simulink model "PMSM_FOC_CascadeControl"  (R2026a)
settings: Solver=ode4  StopTime=simulation_stop_time_s  FixedStep=Ts_current
InitFcn:
  | init_pmsm_foc_cascade
values from neighbouring files (symbols this model uses):
  iq_ref_limit_a = 8.0    (= 8)    [init_pmsm_foc_cascade.m]
  Ki_id = 300.0    (= 300)    [init_pmsm_foc_cascade.m]
  Ki_iq = 300.0    (= 300)    [init_pmsm_foc_cascade.m]
  Ki_speed = 4.0    (= 4)    [init_pmsm_foc_cascade.m]
  Kp_id = 1.5    [init_pmsm_foc_cascade.m]
  Kp_iq = 1.5    [init_pmsm_foc_cascade.m]
  Kp_position = 8.0    (= 8)    [init_pmsm_foc_cascade.m]
  Kp_speed = 0.20    (= 0.2)    [init_pmsm_foc_cascade.m]
  load_torque_nm = 0.0    (= 0)    [init_pmsm_foc_cascade.m]
  pmsm_B_nms = 1.0e-5    (= 1e-05)    [init_pmsm_foc_cascade.m]
  pmsm_flux_wb = 6.0e-3    (= 0.006)    [init_pmsm_foc_cascade.m]
  pmsm_J_kg_m2 = 2.0e-5    (= 2e-05)    [init_pmsm_foc_cascade.m]
  pmsm_Ld_h = 2.0e-4    (= 0.0002)    [init_pmsm_foc_cascade.m]
  pmsm_Lq_h = 2.0e-4    (= 0.0002)    [init_pmsm_foc_cascade.m]
  pmsm_pole_pairs = 7    [init_pmsm_foc_cascade.m]
  pmsm_Rs_ohm = 0.30    (= 0.3)    [init_pmsm_foc_cascade.m]
  position_step_time_s = 0.02    [init_pmsm_foc_cascade.m]
  speed_ref_limit_rad_s = 80.0    (= 80)    [init_pmsm_foc_cascade.m]
  Ts_current = 1.0e-4    (= 0.0001)    [init_pmsm_foc_cascade.m]
  Ts_position = Ts_current    (= 0.0001)    [init_pmsm_foc_cascade.m]
  Ts_speed = Ts_current    (= 0.0001)    [init_pmsm_foc_cascade.m]
  Vdc = 12.0    (= 12)    [init_pmsm_foc_cascade.m]
  voltage_limit_v = Vdc / sqrt(3.0)    [init_pmsm_foc_cascade.m]
libraries: slpidlib x3
settings Model: Creator=tgs27  LastModifiedBy=tgs27

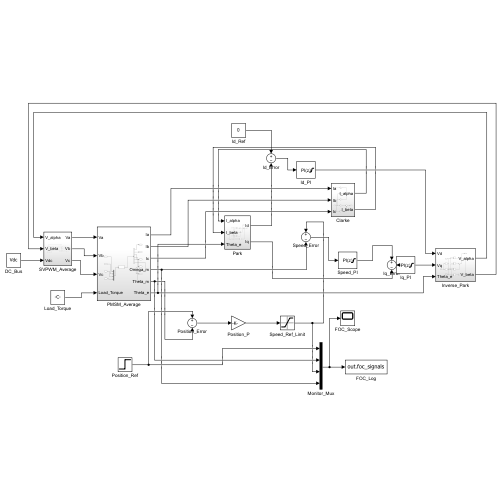
[thumbnail: Simulink's stored preview of the top-level diagram]
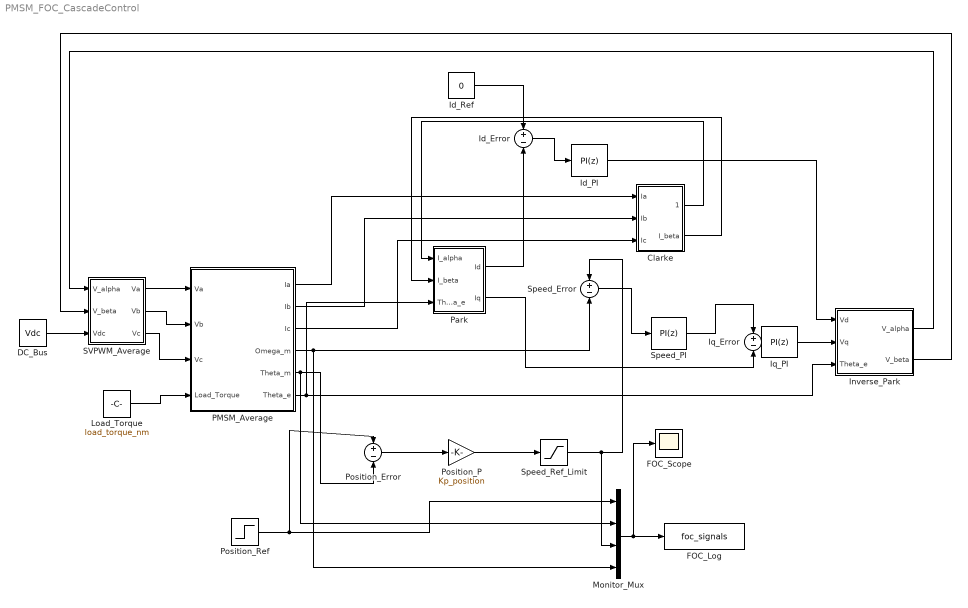
== system PMSM_FOC_CascadeControl ==
  Clarke : Subsystem
  DC_Bus : Constant  Value=Vdc
  FOC_Log : ToWorkspace  VariableName=foc_signals  SaveFormat=Structure With Time
  FOC_Scope : Scope
  Id_Error : Sum  Inputs=+-
  Id_PI : slpidlib/PID Controller  Controller=PI  Form=Parallel  TimeDomain=Discrete-time  UseExternalTs=off  SampleTime=Ts_current  IntegratorMethod=Forward Euler  FilterMethod=Forward Euler  ControllerParametersSource=internal  P=Kp_id  I=Ki_id  UseKiTs=off  D=0  UseExternalDerivativeSource=off  N=100  UseFilter=on  TunerSelectOption=Transfer Function Based (PID Tuner App)  InitialConditionSource=internal  InitialConditionForIntegrator=0  InitialConditionForFilter=0  DifferentiatorICPrevScaledInput=0  ExternalReset=none  TrackingMode=off  Kt=1  LimitOutput=on  SatLimitsSource=internal  UpperSaturationLimit=voltage_limit_v  LowerSaturationLimit=-voltage_limit_v  LinearizeAsGain=on  AntiWindupMode=none  Kb=1  LimitIntegrator=off  UpperIntegratorSaturationLimit=inf  LowerIntegratorSaturationLimit=-inf  POutMin=[]  POutMax=[]  IOutMin=[]  IOutMax=[]  DOutMin=[]  DOutMax=[]  NOutMin=[]  NOutMax=[]  SumOutMin=[]  SumOutMax=[]  SaturationOutMin=[]  SaturationOutMax=[]  PParamMin=[]  PParamMax=[]  IParamMin=[]  IParamMax=[]  DParamMin=[]  DParamMax=[]  NParamMin=[]  NParamMax=[]  KbParamMin=[]  KbParamMax=[]  KtParamMin=[]  KtParamMax=[]  KbOutMin=[]  KbOutMax=[]  KtOutMin=[]  KtOutMax=[]  IntegratorOutMin=[]  IntegratorOutMax=[]  FilterOutMin=[]  FilterOutMax=[]  SumI1OutMin=[]  SumI1OutMax=[]  SumI2OutMin=[]  SumI2OutMax=[]  SumI3OutMin=[]  SumI3OutMax=[]  SumI4OutMin=[]  SumI4OutMax=[]  SumDOutMin=[]  SumDOutMax=[]  DifferentiatorOutMin=[]  DifferentiatorOutMax=[]  FilterDiffOutCoefMin=[]  FilterDiffOutCoefMax=[]  ReciprocalOutMin=[]  ReciprocalOutMax=[]  SumDenOutMin=[]  SumDenOutMax=[]  SumNumOutMin=[]  SumNumOutMax=[]  DivideOutMin=[]  DivideOutMax=[]  UdiffTsProdOutMin=[]  UdiffTsProdOutMax=[]  NTsProdOutMin=[]  NTsProdOutMax=[]  UintegralTsProdOutMin=[]  UintegralTsProdOutMax=[]  UngainTsProdOutMin=[]  UngainTsProdOutMax=[]  ClampingZeroOutDataTypeStr=Inherit: Inherit via back propagation  ClampingZeroOutMin=[]  ClampingZeroOutMax=[]  FilterDenConstantOutDataTypeStr=Inherit: Inherit via back propagation  FilterDenConstantOutMin=[]  FilterDenConstantOutMax=[]  PCopyOutDataTypeStr=Inherit: Inherit via back propagation  PCopyOutMin=[]  PCopyOutMax=[]  NCopyOutDataTypeStr=Inherit: Inherit via back propagation  NCopyOutMin=[]  NCopyOutMax=[]  IntegratorContinuousStateAttributes=''  IntegratorStateMustResolveToSignalObject=off  IntegratorRTWStateStorageClass=Auto  FilterContinuousStateAttributes=''  FilterStateMustResolveToSignalObject=off  FilterRTWStateStorageClass=Auto  ParallelPVariant=InternalParameters  IdealPVariant=Disabled  IVariant=InternalParameters  DVariant=Disabled  IntegratorVariant=Discrete  SatVariant=Enabled  AWVariant=Passthrough  PCopyVariant=Disabled  TRVariant=Disabled  FdbkBlocksVariant=Forward  IdealPFdbkVariant=Disabled  SatFdbkVariant=Disabled  DerivativeFilterVariant=Disabled  NVariant=Disabled  NCopyVariant=Disabled_SignalSpec  FilterICVariant=Disabled  IntegratorICVariant=InternalICs  ExternalResetVariant=Disabled  TRSumVariant=Passthrough  SumFdbkVariant=Disabled  SumVariant=Sum_PI  TsampFilterVariant=InternalTs  TsampNgainVariant=Passthrough  TsampIntegralVariant=Disabled_SignalSpec  ExternalSaturationOutDataTypeStr=Inherit: Same as second input  DerivativeSourceVariant=Disabled  PreIntVariant=InternalPreInt
  Id_Ref : Constant  Value=0
  Inverse_Park : Subsystem
  Iq_Error : Sum  Inputs=+-
  Iq_PI : slpidlib/PID Controller  Controller=PI  Form=Parallel  TimeDomain=Discrete-time  UseExternalTs=off  SampleTime=Ts_current  IntegratorMethod=Forward Euler  FilterMethod=Forward Euler  ControllerParametersSource=internal  P=Kp_iq  I=Ki_iq  UseKiTs=off  D=0  UseExternalDerivativeSource=off  N=100  UseFilter=on  TunerSelectOption=Transfer Function Based (PID Tuner App)  InitialConditionSource=internal  InitialConditionForIntegrator=0  InitialConditionForFilter=0  DifferentiatorICPrevScaledInput=0  ExternalReset=none  TrackingMode=off  Kt=1  LimitOutput=on  SatLimitsSource=internal  UpperSaturationLimit=voltage_limit_v  LowerSaturationLimit=-voltage_limit_v  LinearizeAsGain=on  AntiWindupMode=none  Kb=1  LimitIntegrator=off  UpperIntegratorSaturationLimit=inf  LowerIntegratorSaturationLimit=-inf  POutMin=[]  POutMax=[]  IOutMin=[]  IOutMax=[]  DOutMin=[]  DOutMax=[]  NOutMin=[]  NOutMax=[]  SumOutMin=[]  SumOutMax=[]  SaturationOutMin=[]  SaturationOutMax=[]  PParamMin=[]  PParamMax=[]  IParamMin=[]  IParamMax=[]  DParamMin=[]  DParamMax=[]  NParamMin=[]  NParamMax=[]  KbParamMin=[]  KbParamMax=[]  KtParamMin=[]  KtParamMax=[]  KbOutMin=[]  KbOutMax=[]  KtOutMin=[]  KtOutMax=[]  IntegratorOutMin=[]  IntegratorOutMax=[]  FilterOutMin=[]  FilterOutMax=[]  SumI1OutMin=[]  SumI1OutMax=[]  SumI2OutMin=[]  SumI2OutMax=[]  SumI3OutMin=[]  SumI3OutMax=[]  SumI4OutMin=[]  SumI4OutMax=[]  SumDOutMin=[]  SumDOutMax=[]  DifferentiatorOutMin=[]  DifferentiatorOutMax=[]  FilterDiffOutCoefMin=[]  FilterDiffOutCoefMax=[]  ReciprocalOutMin=[]  ReciprocalOutMax=[]  SumDenOutMin=[]  SumDenOutMax=[]  SumNumOutMin=[]  SumNumOutMax=[]  DivideOutMin=[]  DivideOutMax=[]  UdiffTsProdOutMin=[]  UdiffTsProdOutMax=[]  NTsProdOutMin=[]  NTsProdOutMax=[]  UintegralTsProdOutMin=[]  UintegralTsProdOutMax=[]  UngainTsProdOutMin=[]  UngainTsProdOutMax=[]  ClampingZeroOutDataTypeStr=Inherit: Inherit via back propagation  ClampingZeroOutMin=[]  ClampingZeroOutMax=[]  FilterDenConstantOutDataTypeStr=Inherit: Inherit via back propagation  FilterDenConstantOutMin=[]  FilterDenConstantOutMax=[]  PCopyOutDataTypeStr=Inherit: Inherit via back propagation  PCopyOutMin=[]  PCopyOutMax=[]  NCopyOutDataTypeStr=Inherit: Inherit via back propagation  NCopyOutMin=[]  NCopyOutMax=[]  IntegratorContinuousStateAttributes=''  IntegratorStateMustResolveToSignalObject=off  IntegratorRTWStateStorageClass=Auto  FilterContinuousStateAttributes=''  FilterStateMustResolveToSignalObject=off  FilterRTWStateStorageClass=Auto  ParallelPVariant=InternalParameters  IdealPVariant=Disabled  IVariant=InternalParameters  DVariant=Disabled  IntegratorVariant=Discrete  SatVariant=Enabled  AWVariant=Passthrough  PCopyVariant=Disabled  TRVariant=Disabled  FdbkBlocksVariant=Forward  IdealPFdbkVariant=Disabled  SatFdbkVariant=Disabled  DerivativeFilterVariant=Disabled  NVariant=Disabled  NCopyVariant=Disabled_SignalSpec  FilterICVariant=Disabled  IntegratorICVariant=InternalICs  ExternalResetVariant=Disabled  TRSumVariant=Passthrough  SumFdbkVariant=Disabled  SumVariant=Sum_PI  TsampFilterVariant=InternalTs  TsampNgainVariant=Passthrough  TsampIntegralVariant=Disabled_SignalSpec  ExternalSaturationOutDataTypeStr=Inherit: Same as second input  DerivativeSourceVariant=Disabled  PreIntVariant=InternalPreInt
  Load_Torque : Constant  Value=load_torque_nm
  Monitor_Mux : Mux
  PMSM_Average : Subsystem
  Park : Subsystem
  Position_Error : Sum  Inputs=+-
  Position_P : Gain  Gain=Kp_position
  Position_Ref : Step  Time=position_step_time_s  FinalValue=position_step_rad  SampleTime=Ts_position
  SVPWM_Average : Subsystem
  Speed_Error : Sum  Inputs=+-
  Speed_PI : slpidlib/PID Controller  Controller=PI  Form=Parallel  TimeDomain=Discrete-time  UseExternalTs=off  SampleTime=Ts_speed  IntegratorMethod=Forward Euler  FilterMethod=Forward Euler  ControllerParametersSource=internal  P=Kp_speed  I=Ki_speed  UseKiTs=off  D=0  UseExternalDerivativeSource=off  N=100  UseFilter=on  TunerSelectOption=Transfer Function Based (PID Tuner App)  InitialConditionSource=internal  InitialConditionForIntegrator=0  InitialConditionForFilter=0  DifferentiatorICPrevScaledInput=0  ExternalReset=none  TrackingMode=off  Kt=1  LimitOutput=on  SatLimitsSource=internal  UpperSaturationLimit=iq_ref_limit_a  LowerSaturationLimit=-iq_ref_limit_a  LinearizeAsGain=on  AntiWindupMode=none  Kb=1  LimitIntegrator=off  UpperIntegratorSaturationLimit=inf  LowerIntegratorSaturationLimit=-inf  POutMin=[]  POutMax=[]  IOutMin=[]  IOutMax=[]  DOutMin=[]  DOutMax=[]  NOutMin=[]  NOutMax=[]  SumOutMin=[]  SumOutMax=[]  SaturationOutMin=[]  SaturationOutMax=[]  PParamMin=[]  PParamMax=[]  IParamMin=[]  IParamMax=[]  DParamMin=[]  DParamMax=[]  NParamMin=[]  NParamMax=[]  KbParamMin=[]  KbParamMax=[]  KtParamMin=[]  KtParamMax=[]  KbOutMin=[]  KbOutMax=[]  KtOutMin=[]  KtOutMax=[]  IntegratorOutMin=[]  IntegratorOutMax=[]  FilterOutMin=[]  FilterOutMax=[]  SumI1OutMin=[]  SumI1OutMax=[]  SumI2OutMin=[]  SumI2OutMax=[]  SumI3OutMin=[]  SumI3OutMax=[]  SumI4OutMin=[]  SumI4OutMax=[]  SumDOutMin=[]  SumDOutMax=[]  DifferentiatorOutMin=[]  DifferentiatorOutMax=[]  FilterDiffOutCoefMin=[]  FilterDiffOutCoefMax=[]  ReciprocalOutMin=[]  ReciprocalOutMax=[]  SumDenOutMin=[]  SumDenOutMax=[]  SumNumOutMin=[]  SumNumOutMax=[]  DivideOutMin=[]  DivideOutMax=[]  UdiffTsProdOutMin=[]  UdiffTsProdOutMax=[]  NTsProdOutMin=[]  NTsProdOutMax=[]  UintegralTsProdOutMin=[]  UintegralTsProdOutMax=[]  UngainTsProdOutMin=[]  UngainTsProdOutMax=[]  ClampingZeroOutDataTypeStr=Inherit: Inherit via back propagation  ClampingZeroOutMin=[]  ClampingZeroOutMax=[]  FilterDenConstantOutDataTypeStr=Inherit: Inherit via back propagation  FilterDenConstantOutMin=[]  FilterDenConstantOutMax=[]  PCopyOutDataTypeStr=Inherit: Inherit via back propagation  PCopyOutMin=[]  PCopyOutMax=[]  NCopyOutDataTypeStr=Inherit: Inherit via back propagation  NCopyOutMin=[]  NCopyOutMax=[]  IntegratorContinuousStateAttributes=''  IntegratorStateMustResolveToSignalObject=off  IntegratorRTWStateStorageClass=Auto  FilterContinuousStateAttributes=''  FilterStateMustResolveToSignalObject=off  FilterRTWStateStorageClass=Auto  ParallelPVariant=InternalParameters  IdealPVariant=Disabled  IVariant=InternalParameters  DVariant=Disabled  IntegratorVariant=Discrete  SatVariant=Enabled  AWVariant=Passthrough  PCopyVariant=Disabled  TRVariant=Disabled  FdbkBlocksVariant=Forward  IdealPFdbkVariant=Disabled  SatFdbkVariant=Disabled  DerivativeFilterVariant=Disabled  NVariant=Disabled  NCopyVariant=Disabled_SignalSpec  FilterICVariant=Disabled  IntegratorICVariant=InternalICs  ExternalResetVariant=Disabled  TRSumVariant=Passthrough  SumFdbkVariant=Disabled  SumVariant=Sum_PI  TsampFilterVariant=InternalTs  TsampNgainVariant=Passthrough  TsampIntegralVariant=Disabled_SignalSpec  ExternalSaturationOutDataTypeStr=Inherit: Same as second input  DerivativeSourceVariant=Disabled  PreIntVariant=InternalPreInt
  Speed_Ref_Limit : Saturate  UpperLimit=speed_ref_limit_rad_s  LowerLimit=-speed_ref_limit_rad_s
  wires:
  Position_Ref/1 -> Position_Error/1, Monitor_Mux/1
  PMSM_Average/5(Theta_m) -> Position_Error/2, Monitor_Mux/2
  Position_Error/1 -> Position_P/1
  Position_P/1 -> Speed_Ref_Limit/1
  Speed_Ref_Limit/1 -> Monitor_Mux/3, Speed_Error/1
  PMSM_Average/4(Omega_m) -> Speed_Error/2, Monitor_Mux/4
  Speed_Error/1 -> Speed_PI/1
  Speed_PI/1 -> Iq_Error/1
  Id_Ref/1 -> Id_Error/1
  Park/2(Iq) -> Iq_Error/2
  Iq_Error/1 -> Iq_PI/1
  Park/1(Id) -> Id_Error/2
  Id_Error/1 -> Id_PI/1
  Iq_PI/1 -> Inverse_Park/2(Vq)
  Id_PI/1 -> Inverse_Park/1(Vd)
  PMSM_Average/6(Theta_e) -> Park/3(Theta_e), Inverse_Park/3(Theta_e)
  Inverse_Park/1(V_alpha) -> SVPWM_Average/1(V_alpha)
  Inverse_Park/2(V_beta) -> SVPWM_Average/2(V_beta)
  DC_Bus/1 -> SVPWM_Average/3(Vdc)
  SVPWM_Average/1(Va) -> PMSM_Average/1(Va)
  SVPWM_Average/2(Vb) -> PMSM_Average/2(Vb)
  SVPWM_Average/3(Vc) -> PMSM_Average/3(Vc)
  Load_Torque/1 -> PMSM_Average/4(Load_Torque)
  PMSM_Average/1(Ia) -> Clarke/1(Ia)
  PMSM_Average/2(Ib) -> Clarke/2(Ib)
  PMSM_Average/3(Ic) -> Clarke/3(Ic)
  Clarke/1(I_alpha) -> Park/1(I_alpha)
  Clarke/2(I_beta) -> Park/2(I_beta)
  Monitor_Mux/1 -> FOC_Scope/1, FOC_Log/1

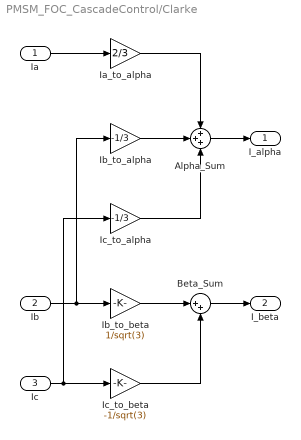
== system PMSM_FOC_CascadeControl/Clarke ==
  Ia : Inport
  Ib : Inport  Port=2
  Ic : Inport  Port=3
  Alpha_Sum : Sum  Inputs=+++
  Beta_Sum : Sum  Inputs=|++
  Ia_to_alpha : Gain  Gain=2/3
  Ib_to_alpha : Gain  Gain=-1/3
  Ib_to_beta : Gain  Gain=1/sqrt(3)
  Ic_to_alpha : Gain  Gain=-1/3
  Ic_to_beta : Gain  Gain=-1/sqrt(3)
  I_alpha : Outport
  I_beta : Outport  Port=2
  wires:
  Beta_Sum/1 -> I_beta/1
  Ic_to_beta/1 -> Beta_Sum/2
  Ib_to_beta/1 -> Beta_Sum/1
  Alpha_Sum/1 -> I_alpha/1
  Ic_to_alpha/1 -> Alpha_Sum/3
  Ib_to_alpha/1 -> Alpha_Sum/2
  Ia_to_alpha/1 -> Alpha_Sum/1
  Ic/1 -> Ic_to_alpha/1, Ic_to_beta/1
  Ib/1 -> Ib_to_alpha/1, Ib_to_beta/1
  Ia/1 -> Ia_to_alpha/1

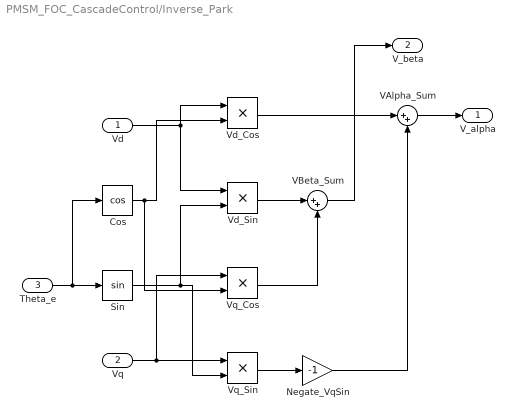
== system PMSM_FOC_CascadeControl/Inverse_Park ==
  Vd : Inport
  Vq : Inport  Port=2
  Theta_e : Inport  Port=3
  Cos : Trigonometry  Operator=cos
  Negate_VqSin : Gain  Gain=-1
  Sin : Trigonometry
  VAlpha_Sum : Sum  Inputs=|++
  VBeta_Sum : Sum  Inputs=|++
  Vd_Cos : Product
  Vd_Sin : Product
  Vq_Cos : Product
  Vq_Sin : Product
  V_alpha : Outport
  V_beta : Outport  Port=2
  wires:
  VBeta_Sum/1 -> V_beta/1
  Vq_Cos/1 -> VBeta_Sum/2
  Vd_Sin/1 -> VBeta_Sum/1
  VAlpha_Sum/1 -> V_alpha/1
  Negate_VqSin/1 -> VAlpha_Sum/2
  Vd_Cos/1 -> VAlpha_Sum/1
  Vq_Sin/1 -> Negate_VqSin/1
  Sin/1 -> Vq_Sin/2, Vd_Sin/2
  Vq/1 -> Vq_Sin/1, Vq_Cos/1
  Cos/1 -> Vd_Cos/2, Vq_Cos/2
  Vd/1 -> Vd_Cos/1, Vd_Sin/1
  Theta_e/1 -> Sin/1, Cos/1

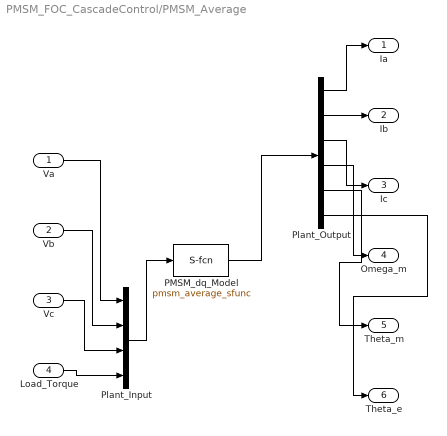
== system PMSM_FOC_CascadeControl/PMSM_Average ==
  Va : Inport
  Vb : Inport  Port=2
  Vc : Inport  Port=3
  Load_Torque : Inport  Port=4
  PMSM_dq_Model : M-S-Function  FunctionName=pmsm_average_sfunc  Parameters=pmsm_pole_pairs,pmsm_Rs_ohm,pmsm_Ld_h,pmsm_Lq_h,pmsm_flux_wb,pmsm_J_kg_m2,pmsm_B_nms
  Plant_Input : Mux
  Plant_Output : Demux  Outputs=6
  Ia : Outport
  Ib : Outport  Port=2
  Ic : Outport  Port=3
  Omega_m : Outport  Port=4
  Theta_m : Outport  Port=5
  Theta_e : Outport  Port=6
  wires:
  Va/1 -> Plant_Input/1
  Vb/1 -> Plant_Input/2
  Vc/1 -> Plant_Input/3
  Load_Torque/1 -> Plant_Input/4
  Plant_Input/1 -> PMSM_dq_Model/1
  PMSM_dq_Model/1 -> Plant_Output/1
  Plant_Output/1 -> Ia/1
  Plant_Output/2 -> Ib/1
  Plant_Output/3 -> Ic/1
  Plant_Output/4 -> Omega_m/1
  Plant_Output/5 -> Theta_m/1
  Plant_Output/6 -> Theta_e/1

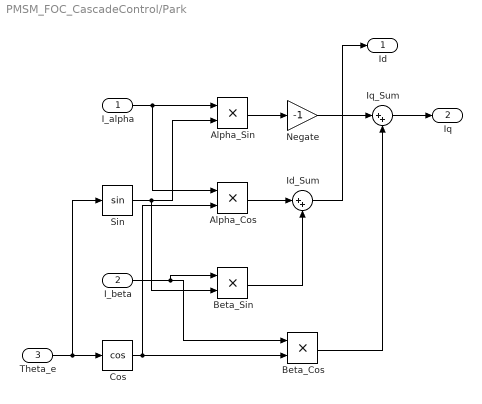
== system PMSM_FOC_CascadeControl/Park ==
  I_alpha : Inport
  I_beta : Inport  Port=2
  Theta_e : Inport  Port=3
  Alpha_Cos : Product
  Alpha_Sin : Product
  Beta_Cos : Product
  Beta_Sin : Product
  Cos : Trigonometry  Operator=cos
  Id_Sum : Sum  Inputs=|++
  Iq_Sum : Sum  Inputs=|++
  Negate : Gain  Gain=-1
  Sin : Trigonometry
  Id : Outport
  Iq : Outport  Port=2
  wires:
  Iq_Sum/1 -> Iq/1
  Beta_Cos/1 -> Iq_Sum/2
  Negate/1 -> Iq_Sum/1
  Alpha_Sin/1 -> Negate/1
  Id_Sum/1 -> Id/1
  Beta_Sin/1 -> Id_Sum/2
  Alpha_Cos/1 -> Id_Sum/1
  Sin/1 -> Beta_Sin/2, Alpha_Sin/2
  I_beta/1 -> Beta_Sin/1, Beta_Cos/1
  Cos/1 -> Alpha_Cos/2, Beta_Cos/2
  I_alpha/1 -> Alpha_Cos/1, Alpha_Sin/1
  Theta_e/1 -> Sin/1, Cos/1

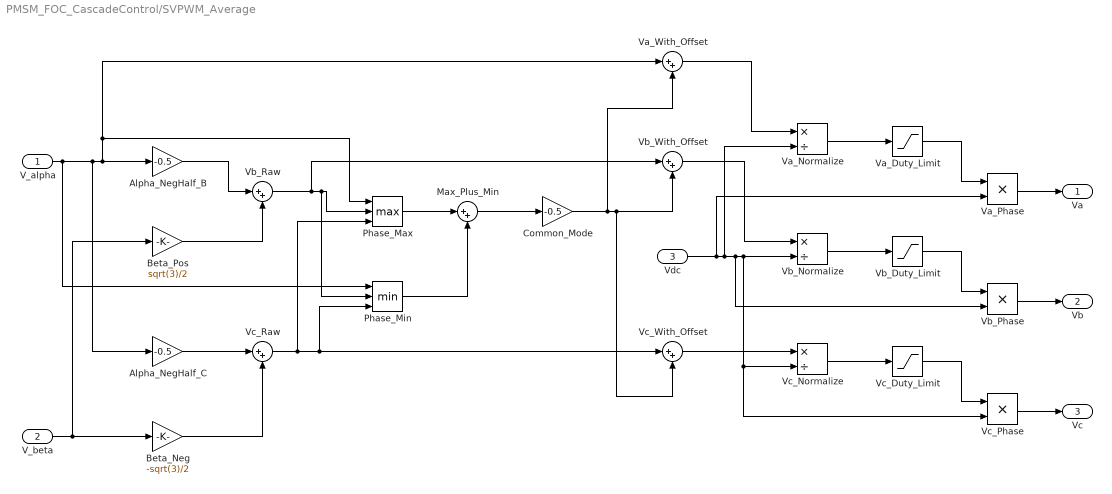
== system PMSM_FOC_CascadeControl/SVPWM_Average ==
  V_alpha : Inport
  V_beta : Inport  Port=2
  Vdc : Inport  Port=3
  Alpha_NegHalf_B : Gain  Gain=-0.5
  Alpha_NegHalf_C : Gain  Gain=-0.5
  Beta_Neg : Gain  Gain=-sqrt(3)/2
  Beta_Pos : Gain  Gain=sqrt(3)/2
  Common_Mode : Gain  Gain=-0.5
  Max_Plus_Min : Sum  Inputs=|++
  Phase_Max : MinMax  Function=max  Inputs=3
  Phase_Min : MinMax  Inputs=3
  Va_Duty_Limit : Saturate
  Va_Normalize : Product  Inputs=*/
  Va_Phase : Product
  Va_With_Offset : Sum  Inputs=|++
  Vb_Duty_Limit : Saturate
  Vb_Normalize : Product  Inputs=*/
  Vb_Phase : Product
  Vb_Raw : Sum  Inputs=|++
  Vb_With_Offset : Sum  Inputs=|++
  Vc_Duty_Limit : Saturate
  Vc_Normalize : Product  Inputs=*/
  Vc_Phase : Product
  Vc_Raw : Sum  Inputs=|++
  Vc_With_Offset : Sum  Inputs=|++
  Va : Outport
  Vb : Outport  Port=2
  Vc : Outport  Port=3
  wires:
  Vc_Phase/1 -> Vc/1
  Vc_Duty_Limit/1 -> Vc_Phase/1
  Vb_Phase/1 -> Vb/1
  Vb_Duty_Limit/1 -> Vb_Phase/1
  Va_Phase/1 -> Va/1
  Va_Duty_Limit/1 -> Va_Phase/1
  Vc_Normalize/1 -> Vc_Duty_Limit/1
  Vb_Normalize/1 -> Vb_Duty_Limit/1
  Va_Normalize/1 -> Va_Duty_Limit/1
  Vc_With_Offset/1 -> Vc_Normalize/1
  Vb_With_Offset/1 -> Vb_Normalize/1
  Vdc/1 -> Vc_Normalize/2, Vc_Phase/2, Vb_Normalize/2, Vb_Phase/2, Va_Normalize/2, Va_Phase/2
  Va_With_Offset/1 -> Va_Normalize/1
  Common_Mode/1 -> Vb_With_Offset/2, Vc_With_Offset/2, Va_With_Offset/2
  Max_Plus_Min/1 -> Common_Mode/1
  Phase_Min/1 -> Max_Plus_Min/2
  Phase_Max/1 -> Max_Plus_Min/1
  Vc_Raw/1 -> Phase_Min/3, Vc_With_Offset/1, Phase_Max/3
  Vb_Raw/1 -> Phase_Max/2, Phase_Min/2, Vb_With_Offset/1
  Beta_Neg/1 -> Vc_Raw/2
  Alpha_NegHalf_C/1 -> Vc_Raw/1
  Beta_Pos/1 -> Vb_Raw/2
  Alpha_NegHalf_B/1 -> Vb_Raw/1
  V_beta/1 -> Beta_Pos/1, Beta_Neg/1
  V_alpha/1 -> Va_With_Offset/1, Phase_Max/1, Alpha_NegHalf_B/1, Alpha_NegHalf_C/1, Phase_Min/1
